simulink model "Simulation_05"  (R2014a)
settings: Solver=ode45  StartTime=0.0  StopTime=10.0  RelTol=1e-3
settings Model: Creator=Dell  LastModifiedBy=Dell

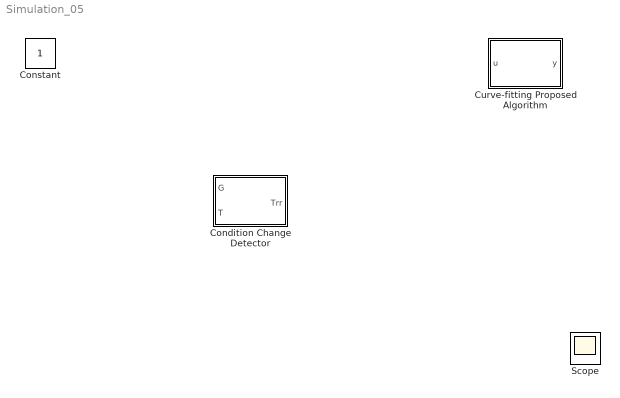
== system Simulation_05 ==
  "Condition Change Detector " : MATLAB Function  TreatAsAtomicUnit=on
  Constant : Constant
  "Curve-fitting Proposed Algorithm " : MATLAB Function  TreatAsAtomicUnit=on
  Scope : Scope

== matlab function Simulation_05/Curve-fitting Proposed Algorithm  ==
  data: u input; y output
function y = fcn(u)
%#codegen

y = u;

== matlab function Simulation_05/Condition Change Detector  ==
  data: G input; Trr output; T input
function Trr = fcn(G, T)

persistent Go To 

Go=G;
To=T;



if 


y = u;
